simulink library "FRN_Library"  (Simulink 7.9)
settings: Solver=VariableStepDiscrete  StartTime=0.0  StopTime=100.0  RelTol=1e-3
libraries: FRN_Library x3, DELS_Library x1
settings Model: Creator=tsprock3  LastModifiedBy=tsprock3

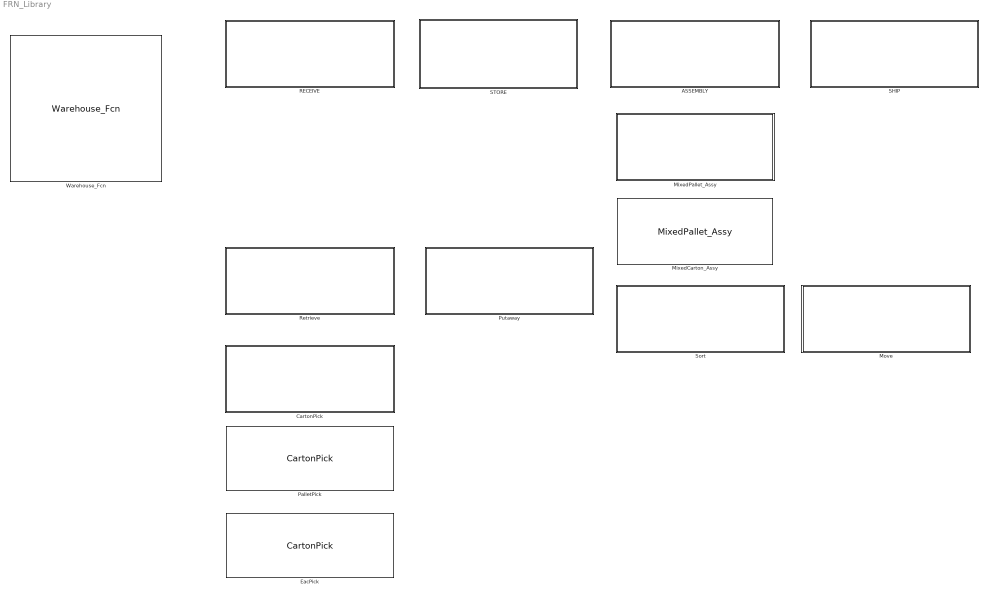
== system FRN_Library ==
  ASSEMBLY : Subsystem
  CartonPick : Subsystem
  EacPick : FRN_Library/CartonPick
  MixedCarton_Assy : FRN_Library/MixedPallet_Assy
  MixedPallet_Assy : Subsystem
  Move : Subsystem
  PalletPick : FRN_Library/CartonPick
  Putaway : Subsystem
  RECEIVE : Subsystem
  Retrieve : Subsystem
  SHIP : Subsystem
  STORE : Subsystem
  Sort : Subsystem
  Warehouse_Fcn : DELS_Library/Warehouse_Fcn

== system FRN_Library/ASSEMBLY ==
  FIFO Queue : FIFOQueue
  N-Server : NServer  NumberOfServers=inf  ServiceTime=0
  Flow_IN : PMIOPort  Port=1  Side=Left
  Message_IN : PMIOPort  Port=2  Side=Left
  Flow_OUT : PMIOPort  Port=3  Side=Right
  Message_OUT : PMIOPort  Port=4  Side=Right
  connections:
  Flow_IN/RConn1 -- FIFO Queue/LConn1
  Flow_OUT/RConn1 -- N-Server/RConn1
  Message_OUT/RConn1 -- Message_IN/RConn1
  FIFO Queue/RConn1 -- N-Server/LConn1

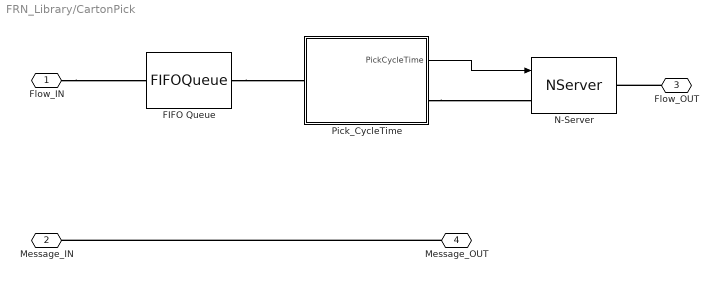
== system FRN_Library/CartonPick ==
  FIFO Queue : FIFOQueue
  N-Server : NServer  NumberOfServers=inf  ServiceTimeFrom=Signal port t  ServiceTime=0
  Pick_CycleTime : Subsystem  mask{pickmean=0, pickstddev=0, traveltime=0}
      mask prompts: pickmean "eachPickMean"; pickstddev "eachPickStdDev"
  Flow_IN : PMIOPort  Port=1  Side=Left
  Message_IN : PMIOPort  Port=2  Side=Left
  Flow_OUT : PMIOPort  Port=3  Side=Right
  Message_OUT : PMIOPort  Port=4  Side=Right
  wires:
  Pick_CycleTime/1(PickCycleTime) -> N-Server/1
  connections:
  Flow_IN/RConn1 -- FIFO Queue/LConn1
  Flow_OUT/RConn1 -- N-Server/RConn1
  Message_OUT/RConn1 -- Message_IN/RConn1
  FIFO Queue/RConn1 -- Pick_CycleTime/LConn1
  Pick_CycleTime/RConn1 -- N-Server/LConn1

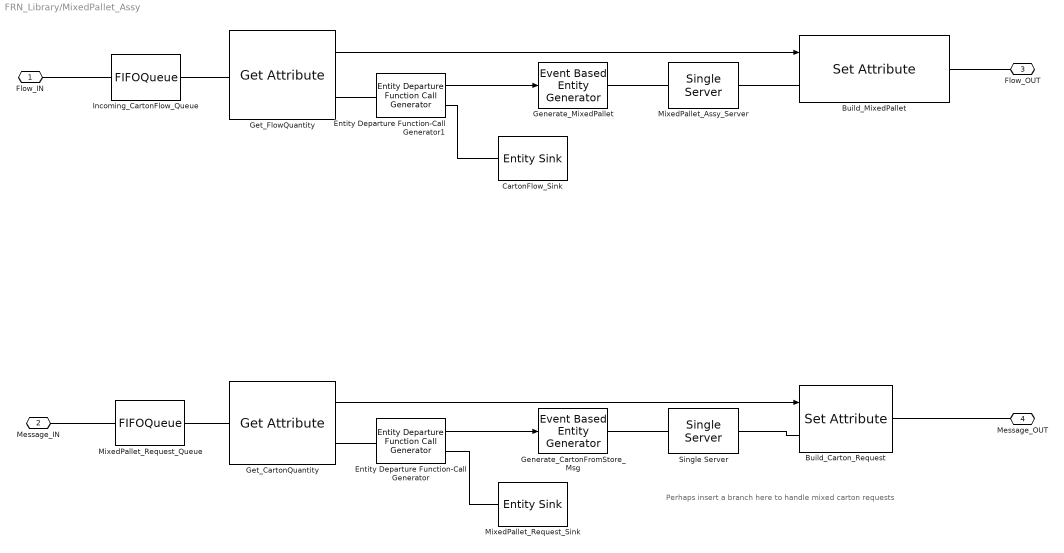
== system FRN_Library/MixedPallet_Assy ==
  note: Perhaps insert a branch here to handle mixed carton requests
  Build_Carton_Request : SetAttribute  AttributeName=UoH|Quantity  AttributeFrom=Dialog|Signal port  AttributeValue=3|1  AttributeTreatAsVector=1|1  EvaluatedAttributeValue={3;[]}
      settings: InputPortMap=u1
  Build_MixedPallet : SetAttribute  AttributeName=UoH|Quantity|CartonQuantity  AttributeFrom=Dialog|Dialog|Signal port  AttributeValue=2|1|1  AttributeTreatAsVector=1|1|1  EvaluatedAttributeValue={2;1;[]}
      settings: InputPortMap=u2
  CartonFlow_Sink : EntitySink
  Entity Departure Function-Call Generator : EntityDepartureFunctionCallGenerator
  Entity Departure Function-Call Generator1 : EntityDepartureFunctionCallGenerator
  Generate_CartonFromStore_Msg : EventBasedEntityGenerator  GenerateEntitiesUpon=Function call from port fcn
  Generate_MixedPallet : EventBasedEntityGenerator  GenerateEntitiesUpon=Function call from port fcn
  Get_CartonQuantity : GetAttribute  AttributeName=CartonQuantity  EvaluatedDefaultAttributeValue={[]}
      settings: OutputPortMap=o1
  Get_FlowQuantity : GetAttribute  AttributeName=Quantity  EvaluatedDefaultAttributeValue={[]}
      settings: OutputPortMap=o1
  Incoming_CartonFlow_Queue : FIFOQueue
  MixedPallet_Assy_Server : SingleServer  ServiceTime=0
  MixedPallet_Request_Queue : FIFOQueue
  MixedPallet_Request_Sink : EntitySink
  Single Server : SingleServer  ServiceTime=0
  Flow_IN : PMIOPort  Port=1  Side=Left
  Message_IN : PMIOPort  Port=2  Side=Left
  Flow_OUT : PMIOPort  Port=3  Side=Right
  Message_OUT : PMIOPort  Port=4  Side=Right
  wires:
  Entity Departure Function-Call Generator/1 -> Generate_CartonFromStore_Msg/1
  Get_CartonQuantity/1 -> Build_Carton_Request/1
  Entity Departure Function-Call Generator1/1 -> Generate_MixedPallet/1
  Get_FlowQuantity/1 -> Build_MixedPallet/1
  connections:
  Flow_IN/RConn1 -- Incoming_CartonFlow_Queue/LConn1
  Message_IN/RConn1 -- MixedPallet_Request_Queue/LConn1
  MixedPallet_Request_Queue/RConn1 -- Get_CartonQuantity/LConn1
  Get_CartonQuantity/RConn1 -- Entity Departure Function-Call Generator/LConn1
  Entity Departure Function-Call Generator/RConn1 -- MixedPallet_Request_Sink/LConn1
  Generate_CartonFromStore_Msg/RConn1 -- Single Server/LConn1
  Single Server/RConn1 -- Build_Carton_Request/LConn1
  Build_Carton_Request/RConn1 -- Message_OUT/RConn1
  Entity Departure Function-Call Generator1/RConn1 -- CartonFlow_Sink/LConn1
  MixedPallet_Assy_Server/RConn1 -- Build_MixedPallet/LConn1
  Generate_MixedPallet/RConn1 -- MixedPallet_Assy_Server/LConn1
  Get_FlowQuantity/RConn1 -- Entity Departure Function-Call Generator1/LConn1
  Incoming_CartonFlow_Queue/RConn1 -- Get_FlowQuantity/LConn1
  Build_MixedPallet/RConn1 -- Flow_OUT/RConn1

== system FRN_Library/Move ==
  FIFO Queue : FIFOQueue
  N-Server : NServer  NumberOfServers=inf  ServiceTime=0
  Flow_IN : PMIOPort  Port=1  Side=Left
  Message_IN : PMIOPort  Port=2  Side=Left
  Flow_OUT : PMIOPort  Port=3  Side=Right
  Message_OUT : PMIOPort  Port=4  Side=Right
  connections:
  Flow_IN/RConn1 -- FIFO Queue/LConn1
  Flow_OUT/RConn1 -- N-Server/RConn1
  Message_OUT/RConn1 -- Message_IN/RConn1
  FIFO Queue/RConn1 -- N-Server/LConn1

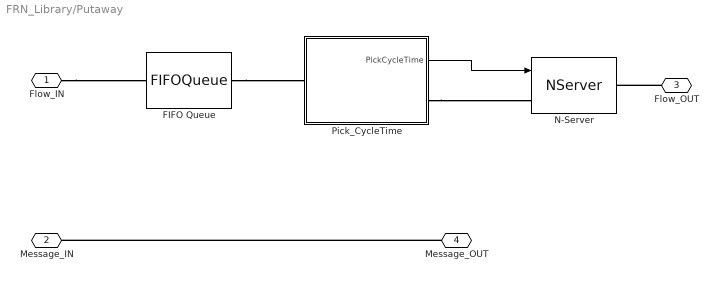
== system FRN_Library/Putaway ==
  FIFO Queue : FIFOQueue
  N-Server : NServer  NumberOfServers=inf  ServiceTimeFrom=Signal port t  ServiceTime=0
  Pick_CycleTime : Subsystem  mask{pickmean=5, pickstddev=0.25, traveltime=80}
      mask prompts: pickmean "eachPickMean"; pickstddev "eachPickStdDev"
  Flow_IN : PMIOPort  Port=1  Side=Left
  Message_IN : PMIOPort  Port=2  Side=Left
  Flow_OUT : PMIOPort  Port=3  Side=Right
  Message_OUT : PMIOPort  Port=4  Side=Right
  wires:
  Pick_CycleTime/1(PickCycleTime) -> N-Server/1
  connections:
  Flow_IN/RConn1 -- FIFO Queue/LConn1
  Flow_OUT/RConn1 -- N-Server/RConn1
  Message_OUT/RConn1 -- Message_IN/RConn1
  FIFO Queue/RConn1 -- Pick_CycleTime/LConn1
  Pick_CycleTime/RConn1 -- N-Server/LConn1

== system FRN_Library/RECEIVE ==
  FIFO Queue : FIFOQueue
  N-Server : NServer  NumberOfServers=inf  ServiceTime=0
  Flow_IN : PMIOPort  Port=1  Side=Left
  Message_IN : PMIOPort  Port=2  Side=Left
  Flow_OUT : PMIOPort  Port=3  Side=Right
  Message_OUT : PMIOPort  Port=4  Side=Right
  connections:
  Flow_IN/RConn1 -- FIFO Queue/LConn1
  Flow_OUT/RConn1 -- N-Server/RConn1
  Message_OUT/RConn1 -- Message_IN/RConn1
  FIFO Queue/RConn1 -- N-Server/LConn1

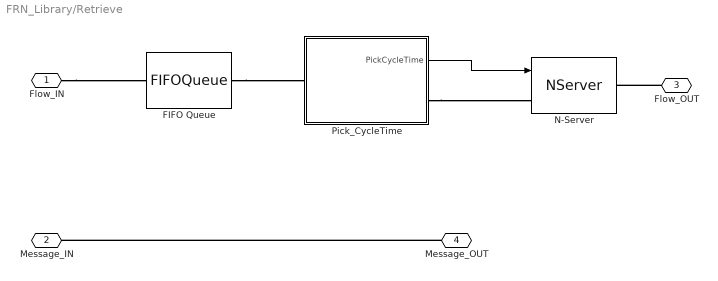
== system FRN_Library/Retrieve ==
  FIFO Queue : FIFOQueue
  N-Server : NServer  NumberOfServers=inf  ServiceTimeFrom=Signal port t  ServiceTime=0
  Pick_CycleTime : Subsystem  mask{pickmean=5, pickstddev=0.25, traveltime=80}
      mask prompts: pickmean "eachPickMean"; pickstddev "eachPickStdDev"
  Flow_IN : PMIOPort  Port=1  Side=Left
  Message_IN : PMIOPort  Port=2  Side=Left
  Flow_OUT : PMIOPort  Port=3  Side=Right
  Message_OUT : PMIOPort  Port=4  Side=Right
  wires:
  Pick_CycleTime/1(PickCycleTime) -> N-Server/1
  connections:
  Flow_IN/RConn1 -- FIFO Queue/LConn1
  Flow_OUT/RConn1 -- N-Server/RConn1
  Message_OUT/RConn1 -- Message_IN/RConn1
  FIFO Queue/RConn1 -- Pick_CycleTime/LConn1
  Pick_CycleTime/RConn1 -- N-Server/LConn1

== system FRN_Library/SHIP ==
  FIFO Queue : FIFOQueue
  N-Server : NServer  NumberOfServers=inf  ServiceTime=0
  Flow_IN : PMIOPort  Port=1  Side=Left
  Message_IN : PMIOPort  Port=2  Side=Left
  Flow_OUT : PMIOPort  Port=3  Side=Right
  Message_OUT : PMIOPort  Port=4  Side=Right
  connections:
  Flow_IN/RConn1 -- FIFO Queue/LConn1
  Flow_OUT/RConn1 -- N-Server/RConn1
  Message_OUT/RConn1 -- Message_IN/RConn1
  FIFO Queue/RConn1 -- N-Server/LConn1

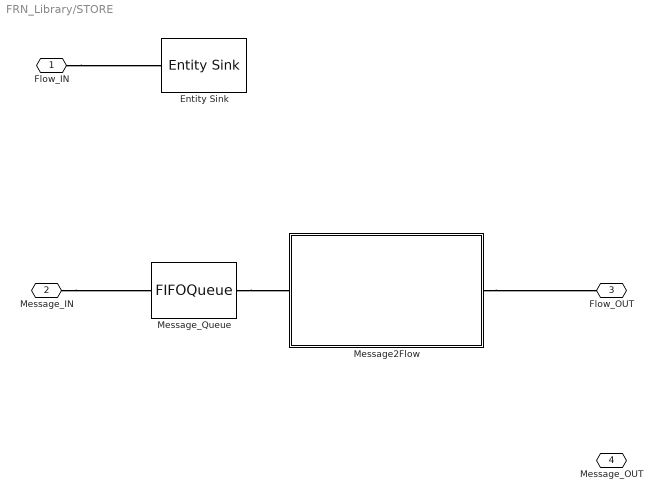
== system FRN_Library/STORE ==
  Entity Sink : EntitySink
  Message2Flow : Subsystem
  Message_Queue : FIFOQueue
  Flow_IN : PMIOPort  Port=1  Side=Left
  Message_IN : PMIOPort  Port=2  Side=Left
  Flow_OUT : PMIOPort  Port=3  Side=Right
  Message_OUT : PMIOPort  Port=4  Side=Right
  connections:
  Flow_IN/RConn1 -- Entity Sink/LConn1
  Message2Flow/RConn1 -- Flow_OUT/RConn1
  Message_IN/RConn1 -- Message_Queue/LConn1
  Message_Queue/RConn1 -- Message2Flow/LConn1

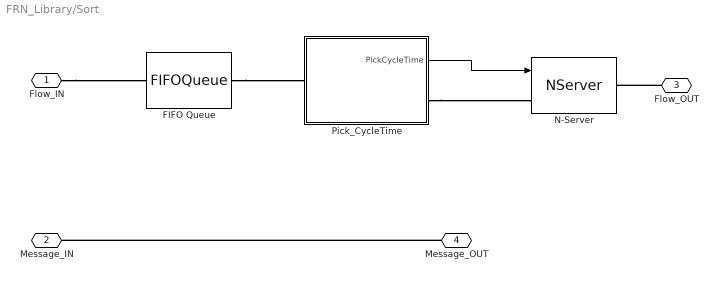
== system FRN_Library/Sort ==
  FIFO Queue : FIFOQueue
  N-Server : NServer  NumberOfServers=inf  ServiceTimeFrom=Signal port t  ServiceTime=0
  Pick_CycleTime : Subsystem  mask{pickmean=5, pickstddev=0.25, traveltime=80}
      mask prompts: pickmean "eachPickMean"; pickstddev "eachPickStdDev"
  Flow_IN : PMIOPort  Port=1  Side=Left
  Message_IN : PMIOPort  Port=2  Side=Left
  Flow_OUT : PMIOPort  Port=3  Side=Right
  Message_OUT : PMIOPort  Port=4  Side=Right
  wires:
  Pick_CycleTime/1(PickCycleTime) -> N-Server/1
  connections:
  Flow_IN/RConn1 -- FIFO Queue/LConn1
  Flow_OUT/RConn1 -- N-Server/RConn1
  Message_OUT/RConn1 -- Message_IN/RConn1
  FIFO Queue/RConn1 -- Pick_CycleTime/LConn1
  Pick_CycleTime/RConn1 -- N-Server/LConn1

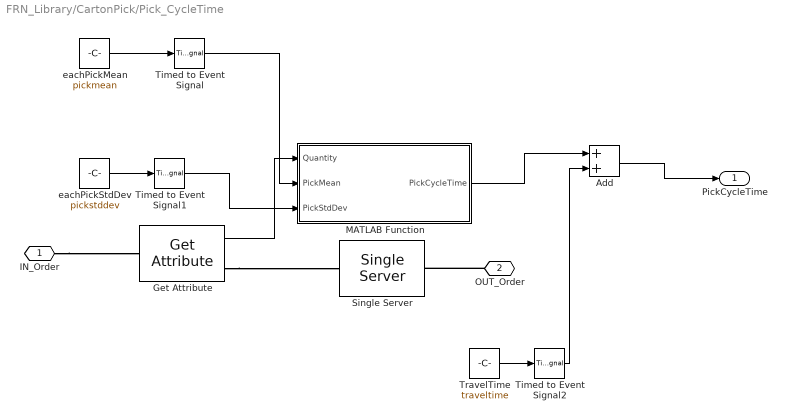
== system FRN_Library/CartonPick/Pick_CycleTime ==
  Add : Sum
  Get Attribute : GetAttribute  AttributeName=Quantity  EvaluatedDefaultAttributeValue={[]}
      settings: OutputPortMap=o1
  MATLAB Function : MATLAB Function  TreatAsAtomicUnit=on
  Single Server : SingleServer  ServiceTime=0
  Timed to Event Signal : TimedToEventSignal
  Timed to Event Signal1 : TimedToEventSignal
  Timed to Event Signal2 : TimedToEventSignal
  TravelTime : Constant  Value=traveltime
  eachPickMean : Constant  Value=pickmean
  eachPickStdDev : Constant  Value=pickstddev
  IN_Order : PMIOPort  Port=1  Side=Left
  OUT_Order : PMIOPort  Port=2  Side=Right
  PickCycleTime : Outport
  wires:
  Get Attribute/1 -> MATLAB Function/1(Quantity)
  MATLAB Function/1(PickCycleTime) -> Add/1
  Add/1 -> PickCycleTime/1
  eachPickStdDev/1 -> Timed to Event Signal1/1
  Timed to Event Signal1/1 -> MATLAB Function/3(PickStdDev)
  eachPickMean/1 -> Timed to Event Signal/1
  Timed to Event Signal/1 -> MATLAB Function/2(PickMean)
  TravelTime/1 -> Timed to Event Signal2/1
  Timed to Event Signal2/1 -> Add/2
  connections:
  Get Attribute/RConn1 -- Single Server/LConn1
  IN_Order/RConn1 -- Get Attribute/LConn1
  OUT_Order/RConn1 -- Single Server/RConn1

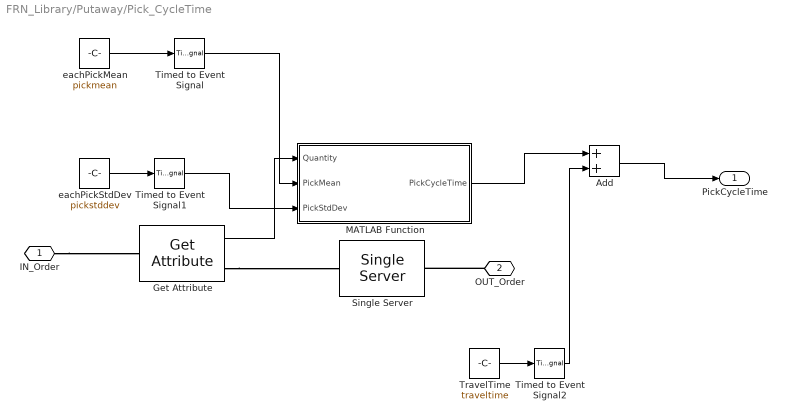
== system FRN_Library/Putaway/Pick_CycleTime ==
  Add : Sum
  Get Attribute : GetAttribute  AttributeName=Carton_Quantity_Layer3  EvaluatedDefaultAttributeValue={[]}
      settings: OutputPortMap=o1
  MATLAB Function : MATLAB Function  TreatAsAtomicUnit=on
  Single Server : SingleServer  ServiceTime=0
  Timed to Event Signal : TimedToEventSignal
  Timed to Event Signal1 : TimedToEventSignal
  Timed to Event Signal2 : TimedToEventSignal
  TravelTime : Constant  Value=traveltime
  eachPickMean : Constant  Value=pickmean
  eachPickStdDev : Constant  Value=pickstddev
  IN_Order : PMIOPort  Port=1  Side=Left
  OUT_Order : PMIOPort  Port=2  Side=Right
  PickCycleTime : Outport
  wires:
  Get Attribute/1 -> MATLAB Function/1(Quantity)
  MATLAB Function/1(PickCycleTime) -> Add/1
  Add/1 -> PickCycleTime/1
  eachPickStdDev/1 -> Timed to Event Signal1/1
  Timed to Event Signal1/1 -> MATLAB Function/3(PickStdDev)
  eachPickMean/1 -> Timed to Event Signal/1
  Timed to Event Signal/1 -> MATLAB Function/2(PickMean)
  TravelTime/1 -> Timed to Event Signal2/1
  Timed to Event Signal2/1 -> Add/2
  connections:
  Get Attribute/RConn1 -- Single Server/LConn1
  IN_Order/RConn1 -- Get Attribute/LConn1
  OUT_Order/RConn1 -- Single Server/RConn1

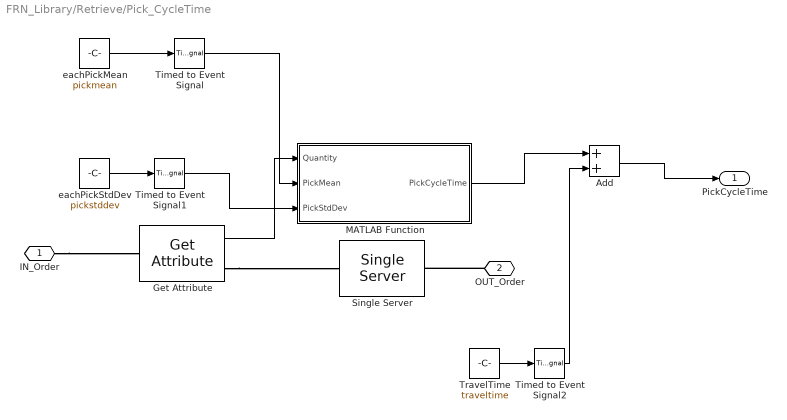
== system FRN_Library/Retrieve/Pick_CycleTime ==
  Add : Sum
  Get Attribute : GetAttribute  AttributeName=Carton_Quantity_Layer3  EvaluatedDefaultAttributeValue={[]}
      settings: OutputPortMap=o1
  MATLAB Function : MATLAB Function  TreatAsAtomicUnit=on
  Single Server : SingleServer  ServiceTime=0
  Timed to Event Signal : TimedToEventSignal
  Timed to Event Signal1 : TimedToEventSignal
  Timed to Event Signal2 : TimedToEventSignal
  TravelTime : Constant  Value=traveltime
  eachPickMean : Constant  Value=pickmean
  eachPickStdDev : Constant  Value=pickstddev
  IN_Order : PMIOPort  Port=1  Side=Left
  OUT_Order : PMIOPort  Port=2  Side=Right
  PickCycleTime : Outport
  wires:
  Get Attribute/1 -> MATLAB Function/1(Quantity)
  MATLAB Function/1(PickCycleTime) -> Add/1
  Add/1 -> PickCycleTime/1
  eachPickStdDev/1 -> Timed to Event Signal1/1
  Timed to Event Signal1/1 -> MATLAB Function/3(PickStdDev)
  eachPickMean/1 -> Timed to Event Signal/1
  Timed to Event Signal/1 -> MATLAB Function/2(PickMean)
  TravelTime/1 -> Timed to Event Signal2/1
  Timed to Event Signal2/1 -> Add/2
  connections:
  Get Attribute/RConn1 -- Single Server/LConn1
  IN_Order/RConn1 -- Get Attribute/LConn1
  OUT_Order/RConn1 -- Single Server/RConn1

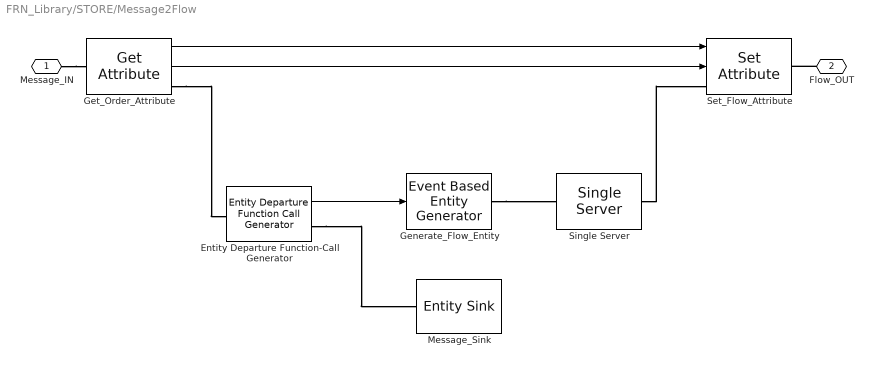
== system FRN_Library/STORE/Message2Flow ==
  Entity Departure Function-Call Generator : EntityDepartureFunctionCallGenerator
  Generate_Flow_Entity : EventBasedEntityGenerator  GenerateEntitiesUpon=Function call from port fcn
  Get_Order_Attribute : GetAttribute  AttributeName=UoH|Quantity  AttributeMissing=Error|Error  AttributeDefaultValue=1|1  AttributeTreatAsVector=1|1  AttributeSendTiming=After entity departure|After entity departure  EvaluatedDefaultAttributeValue={[];[]}
      settings: OutputPortMap=o1,o2
  Message_Sink : EntitySink
  Set_Flow_Attribute : SetAttribute  AttributeName=UoH|Quantity  AttributeFrom=Signal port|Signal port  AttributeValue=1|1  AttributeTreatAsVector=1|1  EvaluatedAttributeValue={[];[]}
      settings: InputPortMap=u0,u1
  Single Server : SingleServer  ServiceTime=0
  Message_IN : PMIOPort  Port=1  Side=Left
  Flow_OUT : PMIOPort  Port=2  Side=Right
  wires:
  Entity Departure Function-Call Generator/1 -> Generate_Flow_Entity/1
  Get_Order_Attribute/1 -> Set_Flow_Attribute/1
  Get_Order_Attribute/2 -> Set_Flow_Attribute/2
  connections:
  Get_Order_Attribute/RConn1 -- Entity Departure Function-Call Generator/LConn1
  Entity Departure Function-Call Generator/RConn1 -- Message_Sink/LConn1
  Generate_Flow_Entity/RConn1 -- Single Server/LConn1
  Single Server/RConn1 -- Set_Flow_Attribute/LConn1
  Message_IN/RConn1 -- Get_Order_Attribute/LConn1
  Flow_OUT/RConn1 -- Set_Flow_Attribute/RConn1

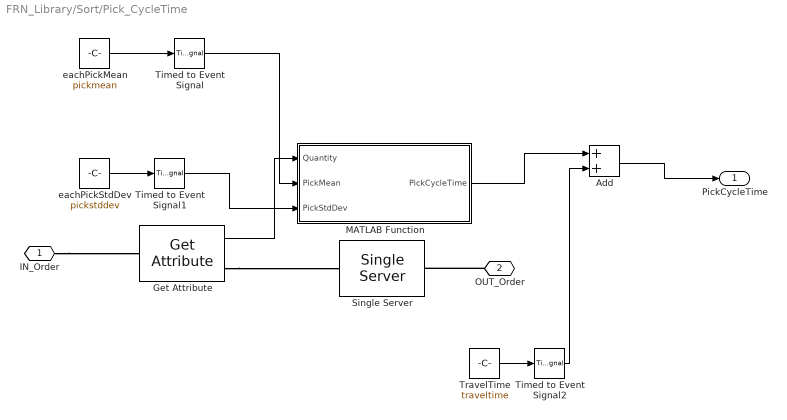
== system FRN_Library/Sort/Pick_CycleTime ==
  Add : Sum
  Get Attribute : GetAttribute  AttributeName=Carton_Quantity_Layer3  EvaluatedDefaultAttributeValue={[]}
      settings: OutputPortMap=o1
  MATLAB Function : MATLAB Function  TreatAsAtomicUnit=on
  Single Server : SingleServer  ServiceTime=0
  Timed to Event Signal : TimedToEventSignal
  Timed to Event Signal1 : TimedToEventSignal
  Timed to Event Signal2 : TimedToEventSignal
  TravelTime : Constant  Value=traveltime
  eachPickMean : Constant  Value=pickmean
  eachPickStdDev : Constant  Value=pickstddev
  IN_Order : PMIOPort  Port=1  Side=Left
  OUT_Order : PMIOPort  Port=2  Side=Right
  PickCycleTime : Outport
  wires:
  Get Attribute/1 -> MATLAB Function/1(Quantity)
  MATLAB Function/1(PickCycleTime) -> Add/1
  Add/1 -> PickCycleTime/1
  eachPickStdDev/1 -> Timed to Event Signal1/1
  Timed to Event Signal1/1 -> MATLAB Function/3(PickStdDev)
  eachPickMean/1 -> Timed to Event Signal/1
  Timed to Event Signal/1 -> MATLAB Function/2(PickMean)
  TravelTime/1 -> Timed to Event Signal2/1
  Timed to Event Signal2/1 -> Add/2
  connections:
  Get Attribute/RConn1 -- Single Server/LConn1
  IN_Order/RConn1 -- Get Attribute/LConn1
  OUT_Order/RConn1 -- Single Server/RConn1

== matlab function Sort/Pick_CycleTime/MATLAB Function ==
  data: Quantity input double; PickCycleTime output double; PickMean input double; PickStdDev input double
function PickCycleTime = fcn(Quantity,  PickMean, PickStdDev)
%#codegen

coder.extrinsic('normrnd');
PickCycleTime = zeros(1, 'double');

Pick_Mean = Quantity*PickMean;
Pick_StdDev =Quantity*PickStdDev;

PickCycleTime = normrnd(Pick_Mean, sqrt(Pick_StdDev));

== matlab function Putaway/Pick_CycleTime/MATLAB Function ==
  data: Quantity input double; PickCycleTime output double; PickMean input double; PickStdDev input double
function PickCycleTime = fcn(Quantity,  PickMean, PickStdDev)
%#codegen

coder.extrinsic('normrnd');
PickCycleTime = zeros(1, 'double');

Pick_Mean = Quantity*PickMean;
Pick_StdDev =Quantity*PickStdDev;

PickCycleTime = normrnd(Pick_Mean, sqrt(Pick_StdDev));

== matlab function Retrieve/Pick_CycleTime/MATLAB Function ==
  data: Quantity input double; PickCycleTime output double; PickMean input double; PickStdDev input double
function PickCycleTime = fcn(Quantity,  PickMean, PickStdDev)
%#codegen

coder.extrinsic('normrnd');
PickCycleTime = zeros(1, 'double');

Pick_Mean = Quantity*PickMean;
Pick_StdDev =Quantity*PickStdDev;

PickCycleTime = normrnd(Pick_Mean, sqrt(Pick_StdDev));

== matlab function CartonPick/Pick_CycleTime/MATLAB Function ==
  data: Quantity input double; PickCycleTime output double; PickMean input double; PickStdDev input double
function PickCycleTime = fcn(Quantity,  PickMean, PickStdDev)
%#codegen

coder.extrinsic('normrnd');
PickCycleTime = zeros(1, 'double');
if eq(Quantity, 0) ==0 
    Pick_Mean = Quantity*PickMean;
    Pick_StdDev =Quantity*PickStdDev;

    PickCycleTime = normrnd(Pick_Mean, sqrt(Pick_StdDev));
end

PickCycleTime = 0;
